simulink model "Lab"  (R2016b)
settings: Solver=VariableStepAuto  StartTime=0.0  StopTime=10.0  RelTol=1e-3
settings Model: Creator=weisched  LastModifiedBy=weisched

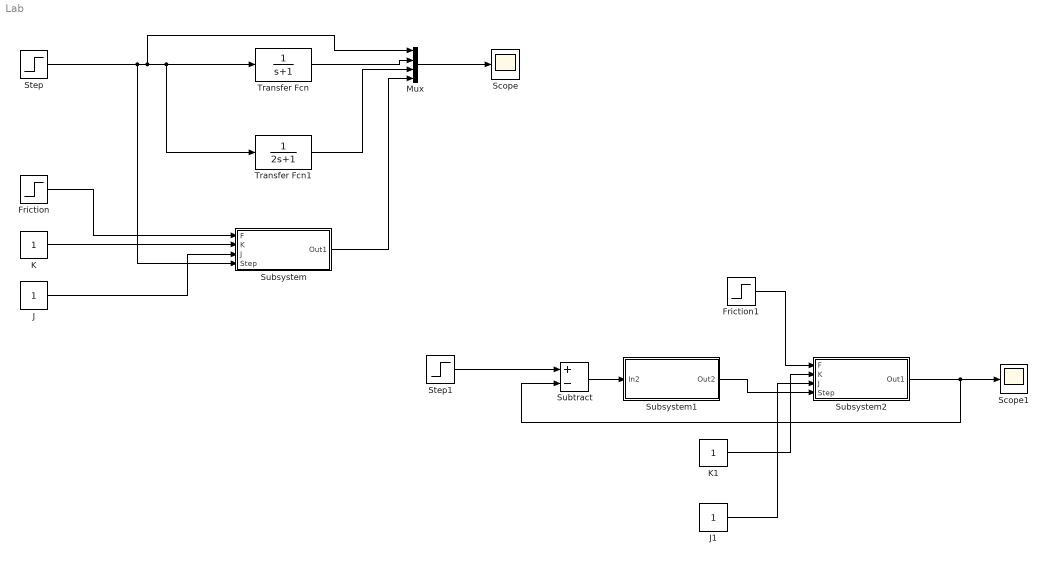
== system Lab ==
  Friction : Step  Time=5  SampleTime=0
  Friction1 : Step  SampleTime=0
  J : Constant
  J1 : Constant
  K : Constant
  K1 : Constant
  Mux : Mux
  Scope : Scope
  Scope1 : Scope
  Step : Step  SampleTime=0
  Step1 : Step  SampleTime=0
  Subsystem : Subsystem
  Subsystem1 : Subsystem
  Subsystem2 : Subsystem
  Subtract : Sum  Inputs=+-
  Transfer Fcn : TransferFcn  Denominator=[1 1]
  Transfer Fcn1 : TransferFcn  Denominator=[2 1]
  wires:
  Step/1 -> Subsystem/4(Step), Mux/1, Transfer Fcn1/1, Transfer Fcn/1
  Transfer Fcn/1 -> Mux/2
  Mux/1 -> Scope/1
  Transfer Fcn1/1 -> Mux/3
  K/1 -> Subsystem/2(K)
  J/1 -> Subsystem/3(J)
  Friction/1 -> Subsystem/1(F)
  Subsystem/1(Out1) -> Mux/4
  Step1/1 -> Subtract/1
  Friction1/1 -> Subsystem2/1(F)
  K1/1 -> Subsystem2/2(K)
  J1/1 -> Subsystem2/3(J)
  Subsystem2/1(Out1) -> Subtract/2, Scope1/1
  Subtract/1 -> Subsystem1/1(In2)
  Subsystem1/1(Out2) -> Subsystem2/4(Step)

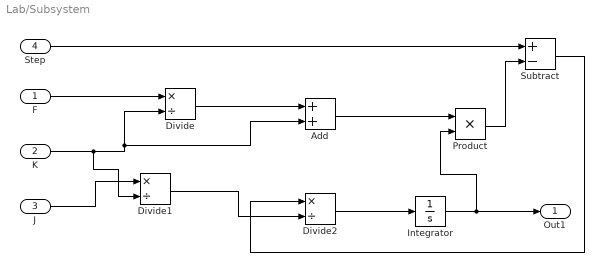
== system Lab/Subsystem ==
  F : Inport
  K : Inport  Port=2
  J : Inport  Port=3
  Step : Inport  Port=4
  Add : Sum
  Divide : Product  Inputs=*/
  Divide1 : Product  Inputs=*/
  Divide2 : Product  Inputs=*/
  Integrator : Integrator
  Product : Product
  Subtract : Sum  Inputs=+-
  Out1 : Outport
  wires:
  F/1 -> Divide/1
  J/1 -> Divide1/1
  K/1 -> Divide1/2, Add/2, Divide/2
  Divide/1 -> Add/1
  Divide1/1 -> Divide2/2
  Add/1 -> Product/1
  Divide2/1 -> Integrator/1
  Integrator/1 -> Product/2, Out1/1
  Product/1 -> Subtract/2
  Step/1 -> Subtract/1
  Subtract/1 -> Divide2/1

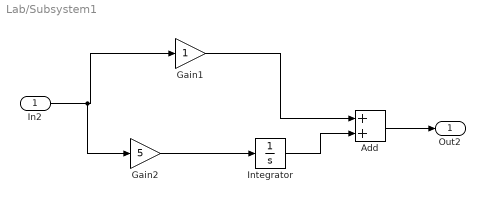
== system Lab/Subsystem1 ==
  In2 : Inport
  Add : Sum
  Gain1 : Gain
  Gain2 : Gain  Gain=5
  Integrator : Integrator
  Out2 : Outport
  wires:
  Gain2/1 -> Integrator/1
  In2/1 -> Gain2/1, Gain1/1
  Add/1 -> Out2/1
  Integrator/1 -> Add/2
  Gain1/1 -> Add/1

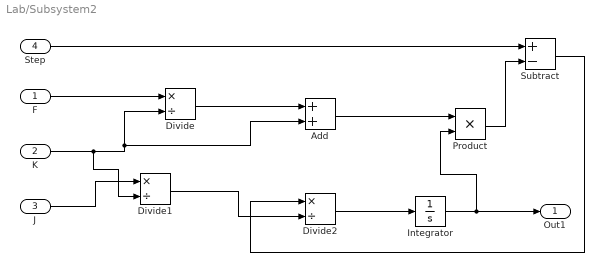
== system Lab/Subsystem2 ==
  F : Inport
  K : Inport  Port=2
  J : Inport  Port=3
  Step : Inport  Port=4
  Add : Sum
  Divide : Product  Inputs=*/
  Divide1 : Product  Inputs=*/
  Divide2 : Product  Inputs=*/
  Integrator : Integrator
  Product : Product
  Subtract : Sum  Inputs=+-
  Out1 : Outport
  wires:
  F/1 -> Divide/1
  J/1 -> Divide1/1
  K/1 -> Divide1/2, Add/2, Divide/2
  Divide/1 -> Add/1
  Divide1/1 -> Divide2/2
  Add/1 -> Product/1
  Divide2/1 -> Integrator/1
  Integrator/1 -> Product/2, Out1/1
  Product/1 -> Subtract/2
  Step/1 -> Subtract/1
  Subtract/1 -> Divide2/1
